simulink model "TestVector"  (Simulink 7.1)
settings: Solver=FixedStepDiscrete  StartTime=0.0  StopTime=10.0  FixedStep=1  RelTol=1e-3
libraries: MPCMdlLib x6
settings Model: Creator=serg  LastModifiedBy=serg

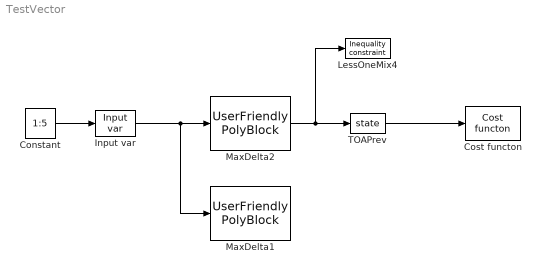
== system TestVector ==
  Constant : Constant  Value=1:5  OutDataType=sfix(16)  OutScaling=2^0
  Cost functon : MPCMdlLib/Cost functon  Tag=OptCost
  Input var : MPCMdlLib/Input var  Tag=OptInput  SystemSampleTime=-1  step_ratio=1  save_name=0
  LessOneMix4 : MPCMdlLib/Inequality constraint  Tag=InequalBlock  CompareSign=> 0
  MaxDelta1 : MPCMdlLib/UserFriendly PolyBlock  Tag=PolyBlock  A=eye(5)  C=2*eye(5)  gA=zeros(1,5)  gC=1  input_type=Vector  output_type=Scalar  port_names=u
  MaxDelta2 : MPCMdlLib/UserFriendly PolyBlock  Tag=PolyBlock  A=eye(5)  C=2*eye(5)  gA=zeros(1,5)  gC=1  input_type=Vector  output_type=Vector  port_names=u
  TOAPrev : MPCMdlLib/state  Tag=OptState  SystemSampleTime=-1  init_val=285  save_name=TOAPrev
  wires:
  Constant/1 -> Input var/1
  MaxDelta2/1 -> TOAPrev/1, LessOneMix4/1
  TOAPrev/1 -> Cost functon/1
  Input var/1 -> MaxDelta2/1, MaxDelta1/1
